simulink model "filter_model"  (R2018a)
settings: Solver=FixedStepDiscrete  StartTime=1.41977e-09  StopTime=3e-06  FixedStep=5e-12  RelTol=1e-3
libraries: powerlib x7
settings Model: Creator=furkan  LastModifiedBy=furkan
settings DataIOCC: ExternalInput=[thirty_noise_signal]

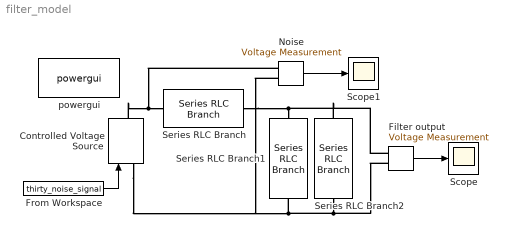
== system filter_model ==
  Controlled Voltage Source : powerlib/Electrical Sources/Controlled Voltage Source  Initialize=on  Source_Type=AC  Amplitude=0  Phase=0  Frequency=0  Measurements=None
  Filter output : powerlib/Measurements/Voltage Measurement  PhasorSimulation=off  OutputType=Complex  PSBequivalent=0
  From Workspace : FromWorkspace  VariableName=thirty_noise_signal  OutDataTypeStr=double  SampleTime=5e-12  Interpolate=off  OutputAfterFinalValue=Setting to zero
  Noise : powerlib/Measurements/Voltage Measurement  PhasorSimulation=off  OutputType=Complex  PSBequivalent=0
  Scope : Scope
  Scope1 : Scope
  Series RLC Branch : powerlib/Elements/Series RLC Branch  LConnTagsString=__new0  RConnTagsString=__new0  BranchType=L  Resistance=1  Inductance=14e-9  SetiL0=off  InitialCurrent=0  Capacitance=1e-6  Setx0=off  InitialVoltage=0  Measurements=None
  Series RLC Branch1 : powerlib/Elements/Series RLC Branch  LConnTagsString=__new0  RConnTagsString=__new0  BranchType=C  Resistance=1  Inductance=14e-9  SetiL0=off  InitialCurrent=0  Capacitance=14e-9  Setx0=off  InitialVoltage=0  Measurements=None
  Series RLC Branch2 : powerlib/Elements/Series RLC Branch  LConnTagsString=__new0  RConnTagsString=__new0  BranchType=R  Resistance=7.96e-09/14e-09  Inductance=14e-9  SetiL0=off  InitialCurrent=0  Capacitance=14e-9  Setx0=off  InitialVoltage=0  Measurements=None
  powergui : powerlib/powergui  Priority=1  SimulationMode=Discrete  SampleTime=5e-12  frequency=60  Iterations=50  frequencyindice=0  Pbase=100e6  ErrMax=1e-4  UnitsV=kV  UnitsW=MW  buscounter=0  FunctionMessages=off  echomessages=off  EnableUseOfTLC=off  CurrentSourceSwitches=off  DisableSnubberDevices=off  DisableRonSwitches=off  DisableVfSwitches=off  DisplayEquations=off  SolverType=Tustin/Backward Euler (TBE)  Interpol=off  ExternalGateDelay=off  methode=off  Ts=100  x0status=blocks  SPID=on  SwTol=0  HookPort=off  RestoreLinks=warning  ResistiveCurrentMeasurement=off  Frange=[0:2:500]  Ylog=off  Xlog=on  ShowGrid=off  save=off  variable=ZData  structure=0  ZoomFFT=off  StartTime=0.0  cycles=1  DisplayStyle=1  fundamental=60  FreqAxis=off  MaxFrequency=1000  frequencyindicesteady=1  RmsSteady=1  display=off
  wires:
  From Workspace/1 -> Controlled Voltage Source/1
  Noise/1 -> Scope1/1
  Filter output/1 -> Scope/1
  connections:
  Controlled Voltage Source/RConn1 -- Noise/LConn1 -- Series RLC Branch/LConn1
  Series RLC Branch/RConn1 -- Filter output/LConn1 -- Series RLC Branch2/LConn1 -- Series RLC Branch1/LConn1
  Series RLC Branch2/RConn1 -- Filter output/LConn2 -- Noise/LConn2 -- Controlled Voltage Source/LConn1 -- Series RLC Branch1/RConn1
